simulink model "trenl"  (Simulink 10.2)
settings: Solver=ode45  StartTime=0.0  StopTime=10.0  RelTol=1e-3  EnableMultiTasking=on
values from neighbouring files (symbols this model uses):
  Am = 15    [lab2var9.m]
  NP = 0.8    [lab2var9.m]
  R = b    [lab2var9.m]
  to = round(rand*100)    [lab2var9.m]
  Ts = 0.001    [lab2var9.m]
libraries: commanapbnd3 x2
settings Model: Creator=mitrofanova  LastModifiedBy=gorbushin_v_a
settings DataIOCC: LimitDataPoints=on  SignalLoggingName=sigsOut
settings OptimizationCC: ExpressionDepthLimit=2147483647  InitFltsAndDblsToZero=on
settings DebuggingCC: SaveWithParameterizedLinksMsg=none  SignalResolutionControl=TryResolveAllWithWarning  MultiTaskDSMMsg=warning  MultiTaskCondExecSysMsg=none  StateNameClashWarn=warning
settings HardwareCC: TargetUnknown=on
settings GRTTargetCC: TargetFcnLib=ansi_tfl_tmw.mat

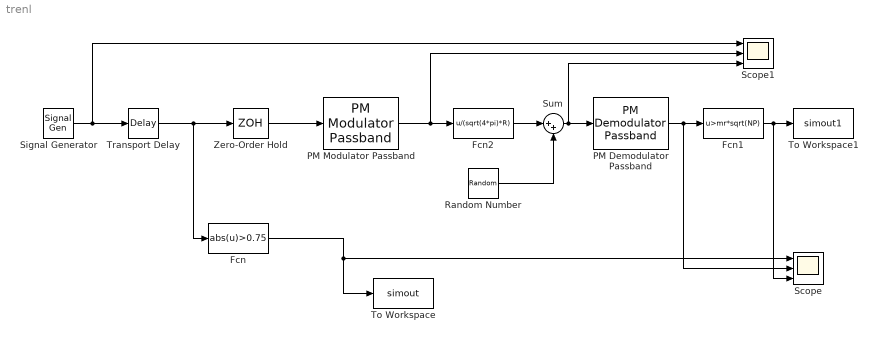
== system trenl ==
  Fcn : Fcn  Expr=abs(u)>0.75  SampleTime=Ts
  Fcn1 : Fcn  Expr=u>mr*sqrt(NP)  SampleTime=Ts
  Fcn2 : Fcn  Expr=u/(sqrt(4*pi)*R)  SampleTime=Ts
  PM Demodulator Passband : commanapbnd3/PM Demodulator Passband  Fc=150  Ph=0  Kc=pi/2  Ho=100
      settings: SourceProductBaseCode=CM
  PM Modulator Passband : commanapbnd3/PM Modulator Passband  Fc=150  Ph=0  Kc=pi/2
      settings: SourceProductBaseCode=CM
  Random Number : RandomNumber  Variance=NP  Seed=to  SampleTime=Ts
  Scope : Scope  NumInputPorts=3
  Scope1 : Scope  NumInputPorts=3
  Signal Generator : SignalGenerator  Amplitude=Am  Units=rad/sec
  Sum : Sum  Inputs=|++  SaturateOnIntegerOverflow=on
  To Workspace : ToWorkspace  VariableName=simout  SampleTime=1
  To Workspace1 : ToWorkspace  VariableName=simout1  SampleTime=1
  Transport Delay : TransportDelay  DelayTime=4.5  BufferSize=10240
  Zero-Order Hold : ZeroOrderHold  SampleTime=Ts
  wires:
  Random Number/1 -> Sum/2
  Fcn/1 -> To Workspace/1, Scope/1
  PM Modulator Passband/1 -> Scope1/2, Fcn2/1
  Fcn2/1 -> Sum/1
  Sum/1 -> PM Demodulator Passband/1, Scope1/3
  PM Demodulator Passband/1 -> Scope/2, Fcn1/1
  Fcn1/1 -> To Workspace1/1, Scope/3
  Signal Generator/1 -> Transport Delay/1, Scope1/1
  Transport Delay/1 -> Zero-Order Hold/1, Fcn/1
  Zero-Order Hold/1 -> PM Modulator Passband/1
